simulink model "magicconst"  (R2016a)
settings: Solver=FixedStepDiscrete  StartTime=0.0  StopTime=10.0  RelTol=1e-3
settings Model: Creator=eruffaldi  LastModifiedBy=eruffaldi

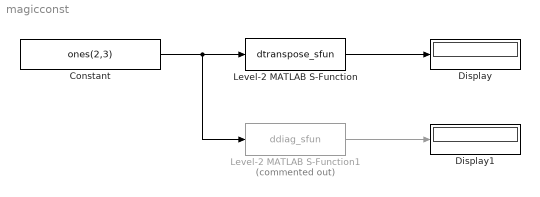
== system magicconst ==
  Constant : Constant  Value=ones(2,3)
  Display : Display
  Display1 : Display
  Level-2 MATLAB S-Function : M-S-Function  FunctionName=dtranspose_sfun
  Level-2 MATLAB S-Function1 : M-S-Function  Commented=on  FunctionName=ddiag_sfun
  wires:
  Constant/1 -> Level-2 MATLAB S-Function1/1, Level-2 MATLAB S-Function/1
  Level-2 MATLAB S-Function/1 -> Display/1
  Level-2 MATLAB S-Function1/1 -> Display1/1
